simulink model "pplaceg_d"  (Simulink 5.0)
settings: Solver=ode23s  StartTime=0.0  StopTime=0.5  RelTol=1e-8  AbsTol=1e-8
values from neighbouring files (symbols this model uses):
  A = [1 -0.43]    [ibm_pp.m]    (also in unstb.m = [1 2 -8])
  B = 0.47    [ibm_pp.m]    (also in unstb.m = [1 -3])
  Ts = 0.01; [B,A,k] = myc2d(G,Ts)    [ant-old.m]    (also in ibm_pp.m = 1; motor_pd.m = 0.25; [B,A,k] = myc2d(G,Ts); unstb.m = 1)
undefined symbols (not defined in the file or in its folder): R, S, TN, zk
settings Model: Creator=kannanm  LastModifiedBy=kannanm  ExtModeAutoUpdateStatusClock=off

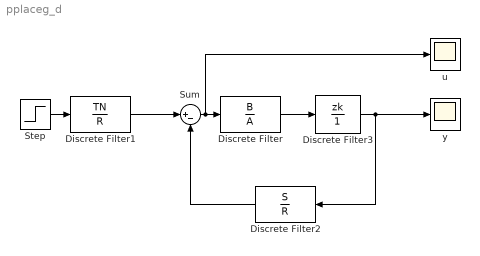
== system pplaceg_d ==
  Discrete Filter : DiscreteFilter  Numerator=B  Denominator=A  SampleTime=Ts
  Discrete Filter1 : DiscreteFilter  Numerator=TN  Denominator=R  SampleTime=Ts
  Discrete Filter2 : DiscreteFilter  Orientation=left  Numerator=S  Denominator=R  SampleTime=Ts
  Discrete Filter3 : DiscreteFilter  Numerator=zk  Denominator=1  SampleTime=Ts
  Step : Step  Time=0  SampleTime=Ts
  Sum : Sum  Inputs=|+-  SaturateOnIntegerOverflow=on
  u : Scope
  y : Scope
  wires:
  Step/1 -> Discrete Filter1/1
  Discrete Filter1/1 -> Sum/1
  Discrete Filter2/1 -> Sum/2
  Discrete Filter3/1 -> y/1, Discrete Filter2/1
  Discrete Filter/1 -> Discrete Filter3/1
  Sum/1 -> Discrete Filter/1, u/1
